simulink model "simu"  (R2024a)
settings: Solver=VariableStepAuto  StartTime=0.0  StopTime=10.0  RelTol=1e-3
undefined symbols (not defined in the file): A, B, h, k1, k2
settings Model: Creator=a2152355  LastModifiedBy=a2152355

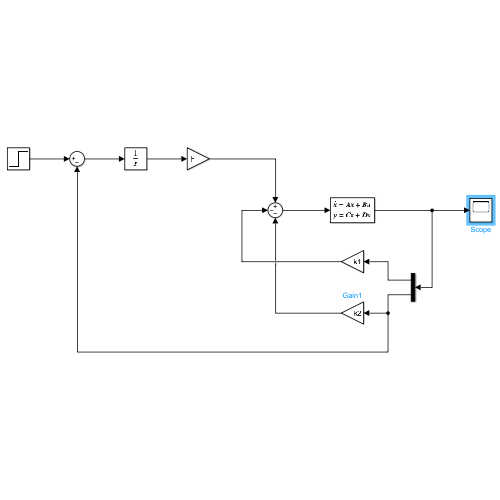
[thumbnail: Simulink's stored preview of the top-level diagram]
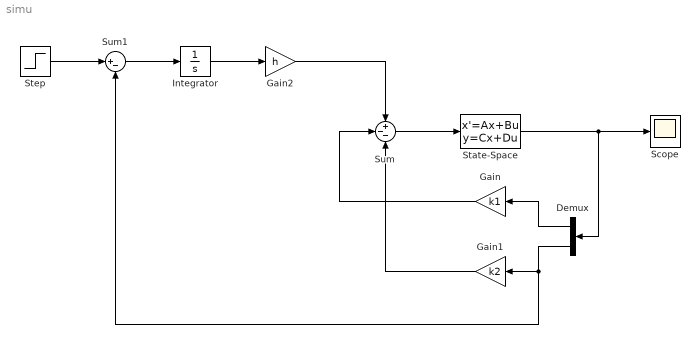
== system simu ==
  Demux : Demux  Outputs=2
  Gain : Gain  Gain=k1
  Gain1 : Gain  Gain=k2
  Gain2 : Gain  Gain=h
  Integrator : Integrator
  Scope : Scope
  State-Space : StateSpace  A=A  B=B  C=eye(2)  D=[0;0]  InitialCondition=[0 0]
  Step : Step  SampleTime=0
  Sum : Sum  Inputs=+--
  Sum1 : Sum  Inputs=|+-
  wires:
  Sum/1 -> State-Space/1
  Gain/1 -> Sum/2
  State-Space/1 -> Scope/1, Demux/1
  Demux/1 -> Gain/1
  Demux/2 -> Gain1/1, Sum1/2
  Gain1/1 -> Sum/3
  Integrator/1 -> Gain2/1
  Step/1 -> Sum1/1
  Sum1/1 -> Integrator/1
  Gain2/1 -> Sum/1
